simulink model "non_linear_observer"  (R2021a)
settings: Solver=VariableStepAuto  StartTime=0.0  StopTime=100  RelTol=1e-3
undefined symbols (not defined in the file): AO, BO, C, CO, DO
settings Model: Creator=savna  LastModifiedBy=savna

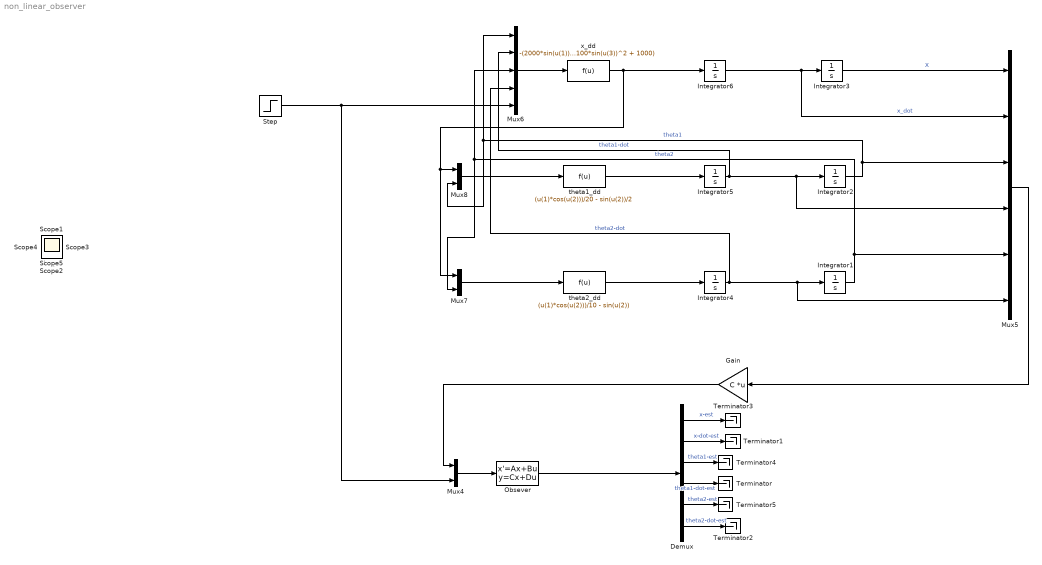
== system non_linear_observer ==
  Demux : Demux  Outputs=6
  Gain : Gain  Gain=C  Multiplication=Matrix(K*u)
  Integrator1 : Integrator  InitialCondition=0.1
  Integrator2 : Integrator  InitialCondition=0.1
  Integrator3 : Integrator  InitialCondition=0.5
  Integrator4 : Integrator
  Integrator5 : Integrator
  Integrator6 : Integrator
  Mux4 : Mux  Inputs=2
  Mux5 : Mux  Inputs=6
  Mux6 : Mux  Inputs=5
  Mux7 : Mux  Inputs=2
  Mux8 : Mux  Inputs=2
  "Obsever " : StateSpace  A=AO  B=BO  C=CO  D=DO  InitialCondition=0
  Step : Step  SampleTime=0
  Terminator{,1..5} (6 alike) : Terminator
  theta1_dd : Fcn  Expr=(u(1)*cos(u(2)))/20 - sin(u(2))/2
  theta2_dd : Fcn  Expr=(u(1)*cos(u(2)))/10 - sin(u(2))
  x_dd : Fcn  Expr=-(2000*sin(u(1))*u(2)^2 + 1000*sin(u(3))*u(4)^2 - u(5) + 1000*cos(u(1))*sin(u(1)) - 1000*cos(u(3))*sin(u(3)))/(100*sin(u(1))^2 + 100*sin(u(3))^2 + 1000)
  Scope{,1..5} (6 alike) : Scope
  wires:
  "Obsever "/1 -> Demux/1
  Demux/2 -> Terminator1/1  "x-dot-est"
  Demux/4 -> Terminator/1  "theta1-dot-est"
  Demux/6 -> Terminator2/1  "theta2-dot-est"
  Step/1 -> Mux6/5, Mux4/2
  Mux4/1 -> "Obsever "/1
  Gain/1 -> Mux4/1
  Integrator2/1 -> Mux8/2, Mux6/1, Mux5/3  "theta1"
  Integrator1/1 -> Mux7/2, Mux6/3, Mux5/5  "theta2"
  theta1_dd/1 -> Integrator5/1
  Mux6/1 -> x_dd/1
  theta2_dd/1 -> Integrator4/1
  Integrator5/1 -> Mux6/2, Mux5/4, Integrator2/1  "theta1-dot"
  x_dd/1 -> Mux7/1, Mux8/1, Integrator6/1
  Mux7/1 -> theta2_dd/1
  Integrator4/1 -> Mux6/4, Integrator1/1, Mux5/6  "theta2-dot"
  Mux8/1 -> theta1_dd/1
  Integrator3/1 -> Mux5/1  "X"
  Integrator6/1 -> Mux5/2, Integrator3/1  "x_dot"
  Mux5/1 -> Gain/1
  Demux/1 -> Terminator3/1  "x-est"
  Demux/3 -> Terminator4/1  "theta1-est"
  Demux/5 -> Terminator5/1  "theta2-est"
